simulink model "feedback_cascade_linearized_sim"  (R2023b)
settings: Solver=VariableStepAuto  StartTime=0.0  StopTime=10.0  RelTol=1e-3
values from neighbouring files (symbols this model uses):
  A1 = bottom_area    (= 2)    [feedback_cascade_precise.m]    (also in lab_7_script.m = 1)
  A2 = bottom_area    (= 2)    [feedback_cascade_precise.m]    (also in lab_7_script.m = 1)
  a_1 = bottom_area * (sqrt(2 * g * (water_level_delta))) / water_level_delta    [feedback_cascade_linearized.m]
  a_2 = bottom_area * (sqrt(2 * g * max_water_level_2)) / max_water_level_2    [feedback_cascade_linearized.m]
  flow_input_step_1 = 0.1 * flow_input_max_1    [feedback_cascade_linearized.m]    (also in feedback_cascade_precise.m)
  flow_input_step_2 = 0    [feedback_cascade_linearized.m]    (also in feedback_cascade_precise.m)
  initial_flow_input_1 = flow_inputs_vec_1(i)    [feedback_cascade_linearized.m]    (also in feedback_cascade_precise.m)
  initial_flow_input_2 = flow_input_max_2    [feedback_cascade_linearized.m]    (also in feedback_cascade_precise.m)
  initial_height_1 = flow_inputs_vec_1(i) / a_1 + initial_height_2    [feedback_cascade_linearized.m]    (also in feedback_cascade_precise.m = 0)
  initial_height_2 = (flow_input_max_2 + initial_flow_input_1) / a_2    [feedback_cascade_linearized.m]    (also in feedback_cascade_precise.m = (         ((flow_input_max_2 + initial_flow_input_1) ^ 2) / )
  T0 = 2    [feedback_cascade_linearized.m]    (also in feedback_cascade_precise.m; lab_7_script.m)
settings Model: Creator=igorkrzywda  LastModifiedBy=igorkrzywda

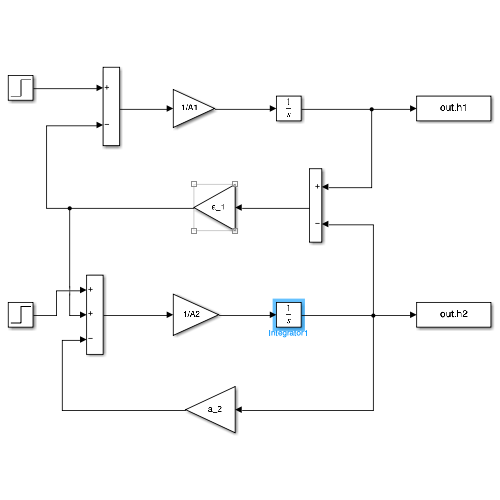
[thumbnail: Simulink's stored preview of the top-level diagram]
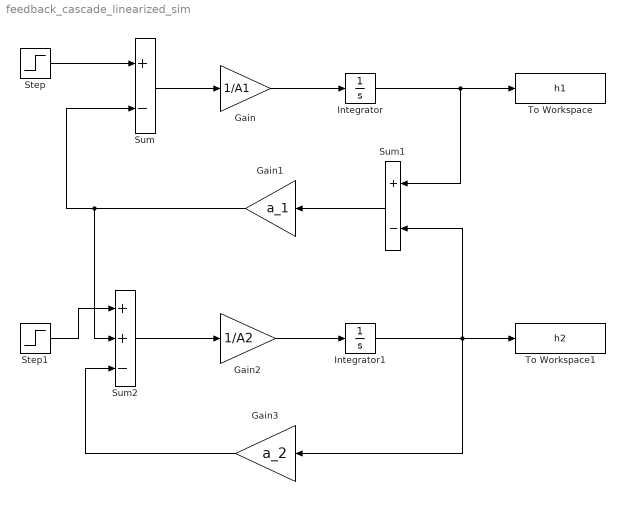
== system feedback_cascade_linearized_sim ==
  Gain : Gain  Gain=1/A1
  Gain1 : Gain  Gain=a_1
  Gain2 : Gain  Gain=1/A2
  Gain3 : Gain  Gain=a_2
  Integrator : Integrator  InitialCondition=initial_height_1
  Integrator1 : Integrator  InitialCondition=initial_height_2
  Step : Step  Time=T0  Before=initial_flow_input_1  After=initial_flow_input_1 + flow_input_step_1  SampleTime=0
  Step1 : Step  Time=T0  Before=initial_flow_input_2  After=initial_flow_input_2 + flow_input_step_2  SampleTime=0
  Sum : Sum  Inputs=+-
  Sum1 : Sum  Inputs=+-
  Sum2 : Sum  Inputs=++-
  To Workspace : ToWorkspace  VariableName=h1  SampleTime=-1
  To Workspace1 : ToWorkspace  VariableName=h2  SampleTime=-1
  wires:
  Step/1 -> Sum/1
  Sum/1 -> Gain/1
  Gain/1 -> Integrator/1
  Integrator/1 -> Sum1/1, To Workspace/1
  Sum1/1 -> Gain1/1
  Gain1/1 -> Sum2/2, Sum/2
  Step1/1 -> Sum2/1
  Sum2/1 -> Gain2/1
  Gain2/1 -> Integrator1/1
  Integrator1/1 -> Gain3/1, To Workspace1/1, Sum1/2
  Gain3/1 -> Sum2/3
